simulink model "UAM_Flight_control"  (R2024b)
settings: Solver=VariableStepAuto  StartTime=0.0  StopTime=10.0  RelTol=1e-3  EnableMultiTasking=on
settings Model: DataDictionary=UAM_data.sldd  Creator=admin  LastModifiedBy=admin
settings SolverCC: PositivePriorityOrder=on
settings OptimizationCC: DefaultParameterBehavior=Inlined  EnhancedBackFolding=on  PassReuseOutputArgsThreshold=0  MaxStackSize=64  OptimizeBlockOrder=speed  DifferentSizesBufferReuse=on  OptimizationCustomize=off
settings DebuggingCC: ParameterTunabilityLossMsg=error
settings ModelReferenceCC: ModelReferenceNumInstancesAllowed=Single
settings SFSimCC: MATLABDynamicMemAlloc=off
settings RTWCC: Description=Create Visual C/C++ Solution File for Simulink Coder  TemplateMakefile=RTW.MSVCBuild
settings CodeAppCC: ForceParamTrailComments=on  OperatorAnnotations=on
settings GRTTargetCC: TargetLangStandard=C89/C90 (ANSI)

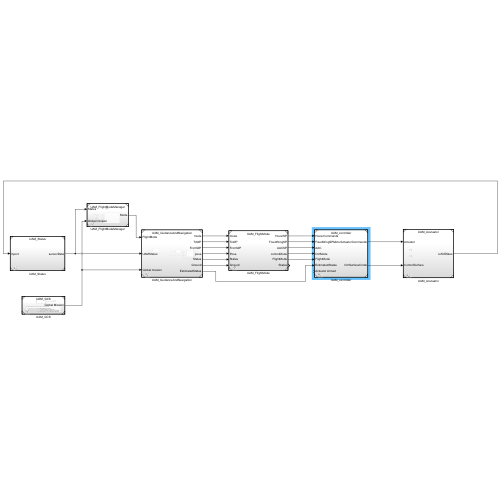
[thumbnail: Simulink's stored preview of the top-level diagram]
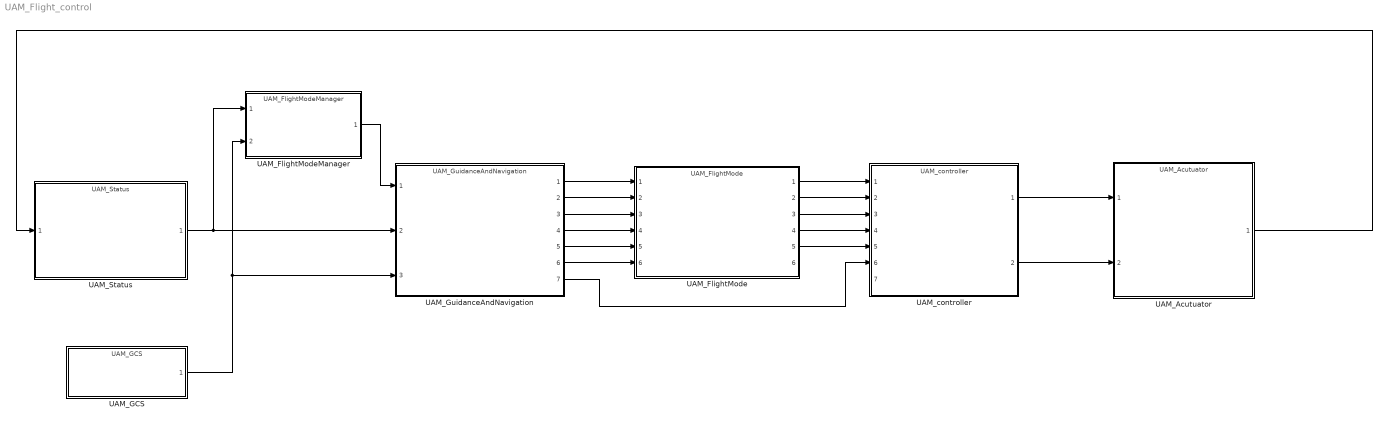
== system UAM_Flight_control ==
  UAM_Acutuator : ModelReference  ModelNameDialog=UAM_Acutuator.slx  SimulationMode=Normal  ModelReferenceVersion=1.9
  UAM_FlightMode : ModelReference  ModelNameDialog=UAM_FlightMode.slx  SimulationMode=Normal  ModelReferenceVersion=1.57
  UAM_FlightModeManager : ModelReference  ModelNameDialog=UAM_FlightModeManager.slx  SimulationMode=Normal  ModelReferenceVersion=1.15
  UAM_GCS : ModelReference  ModelNameDialog=UAM_GCS.slx  SimulationMode=Normal  ModelReferenceVersion=1.5
  UAM_GuidanceAndNavigation : ModelReference  ModelNameDialog=UAM_GuidanceAndNavigation.slx  SimulationMode=Normal  ModelReferenceVersion=1.65
  UAM_Status : ModelReference  ModelNameDialog=UAM_Status.slx  SimulationMode=Normal  ModelReferenceVersion=1.57
  UAM_controller : ModelReference  ModelNameDialog=UAM_controller.slx  SimulationMode=Normal  ModelReferenceVersion=1.22
  wires:
  UAM_controller/1 -> UAM_Acutuator/1
  UAM_controller/2 -> UAM_Acutuator/2
  UAM_Status/1 -> UAM_GuidanceAndNavigation/2, UAM_FlightModeManager/1
  UAM_Acutuator/1 -> UAM_Status/1
  UAM_GCS/1 -> UAM_FlightModeManager/2, UAM_GuidanceAndNavigation/3
  UAM_GuidanceAndNavigation/1 -> UAM_FlightMode/1
  UAM_GuidanceAndNavigation/2 -> UAM_FlightMode/2
  UAM_GuidanceAndNavigation/3 -> UAM_FlightMode/3
  UAM_GuidanceAndNavigation/4 -> UAM_FlightMode/4
  UAM_GuidanceAndNavigation/5 -> UAM_FlightMode/5
  UAM_GuidanceAndNavigation/6 -> UAM_FlightMode/6
  UAM_FlightModeManager/1 -> UAM_GuidanceAndNavigation/1
  UAM_GuidanceAndNavigation/7 -> UAM_controller/6
  UAM_FlightMode/1 -> UAM_controller/1
  UAM_FlightMode/2 -> UAM_controller/2
  UAM_FlightMode/3 -> UAM_controller/3
  UAM_FlightMode/4 -> UAM_controller/4
  UAM_FlightMode/5 -> UAM_controller/5
